simulink model "ObservadorDeLuenbergerEFiltroDeKalman"  (R2023a)
settings: Solver=VariableStepAuto  StartTime=0.0  StopTime=10  RelTol=1e-3
undefined symbols (not defined in the file): A, B, C, Continuous, R, sigma_v, sigma_w, Time, ts
libraries: ctrlSharedLib x1
settings Model: Creator=Cliente  LastModifiedBy=chris
settings SolverCC: AlgebraicLoopSolver=TrustRegion
settings DebuggingCC: UnconnectedInputMsg=warning  UnconnectedOutputMsg=warning  UnconnectedLineMsg=warning
settings ModelReferenceCC: EnableRefExpFcnMdlSchedulingChecks=on
settings SFSimCC: CustomCodeUndefinedFunction=UseInterfaceOnly

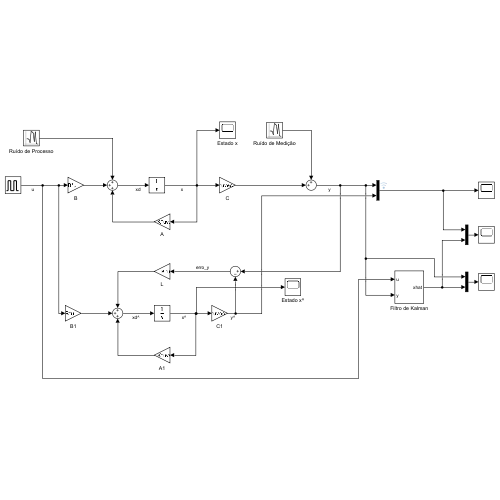
[thumbnail: Simulink's stored preview of the top-level diagram]
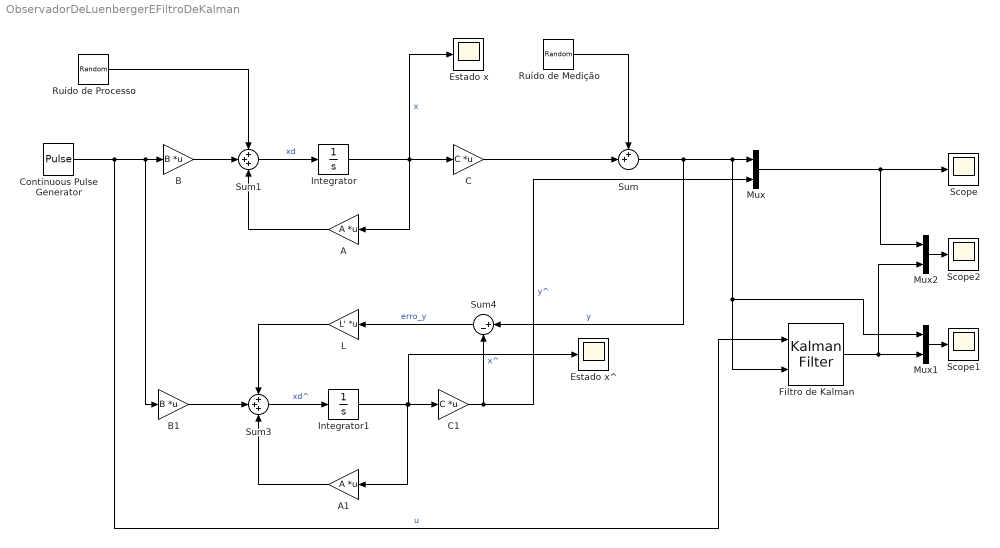
== system ObservadorDeLuenbergerEFiltroDeKalman ==
  A : Gain  Gain=A  Multiplication=Matrix(K*u) (u vector)
  A1 : Gain  Gain=A  Multiplication=Matrix(K*u) (u vector)
  B : Gain  Gain=B  Multiplication=Matrix(K*u)
  B1 : Gain  Gain=B  Multiplication=Matrix(K*u)
  C : Gain  Gain=C  Multiplication=Matrix(K*u) (u vector)
  C1 : Gain  Gain=C  Multiplication=Matrix(K*u) (u vector)
  Continuous Pulse Generator : DiscretePulseGenerator  PulseType=Time based  Amplitude=0.1  Period=1  PulseWidth=50
  Estado x : Scope
  Estado x^ : Scope
  Filtro de Kalman : ctrlSharedLib/Kalman Filter  TimeDomain=Continuous-Time  UseCurrentEstimator=on  ModelSource=Individual A, B, C, D matrices  ModelSourceVariable=ss(0.95,1,1,0,1)  A=A  B=B  C=C  D=0  NumberOfStates=1  NumberOfInputs=1  NumberOfOutputs=1  InitialEstimateSource=Dialog  X0=[0;0]  P0=10  UseK=off  UseGH=off  NumberOfProcessNoiseInputs=1  G=1  TimeInvariantG=on  H=0  TimeInvariantH=on  Q=Q  TimeInvariantQ=on  R=R  TimeInvariantR=on  N=0  TimeInvariantN=on  AddInputPort=on  AddEnablePort=off  OutputEstimatedY=off  OutputP=off  Ts=-1
  Integrator : Integrator  InitialCondition=[0;0]
  Integrator1 : Integrator  InitialCondition=[0;0]
  L : Gain  Gain=L'  Multiplication=Matrix(K*u)
  Mux : Mux  Inputs=2
  Mux1 : Mux  Inputs=2
  Mux2 : Mux  Inputs=2
  Ruído de Medição : RandomNumber  Variance=sigma_v^2  Seed=[23341]  SampleTime=ts
  Ruído de Processo : RandomNumber  Variance=sigma_w^2  Seed=[23341]  SampleTime=ts
  Scope : Scope
  Scope1 : Scope
  Scope2 : Scope
  Sum : Sum  Inputs=++|
  Sum1 : Sum  Inputs=+++
  Sum3 : Sum  Inputs=+++
  Sum4 : Sum  Inputs=|+-
  wires:
  C1/1 -> Mux/2, Sum4/2  "y^"
  B1/1 -> Sum3/2
  Sum3/1 -> Integrator1/1  "xd^"
  Integrator/1 -> Estado x/1, C/1, A/1  "x"
  Sum1/1 -> Integrator/1  "xd"
  A1/1 -> Sum3/3
  Sum4/1 -> L/1  "erro_y"
  Integrator1/1 -> A1/1, C1/1, Estado x^/1  "x^"
  L/1 -> Sum3/1
  A/1 -> Sum1/3
  Ruído de Processo/1 -> Sum1/1
  B/1 -> Sum1/2
  C/1 -> Sum/2
  Ruído de Medição/1 -> Sum/1
  Sum/1 -> Sum4/1, Mux1/1, Filtro de Kalman/2, Mux/1  "y"
  Mux1/1 -> Scope1/1
  Filtro de Kalman/1 -> Mux2/2, Mux1/2
  Continuous Pulse Generator/1 -> Filtro de Kalman/1, B1/1, B/1  "u"
  Mux/1 -> Mux2/1, Scope/1
  Mux2/1 -> Scope2/1
